simulink model "nivel3"  (R2018b)
settings: Solver=VariableStepAuto  StartTime=0.0  StopTime=10.0  RelTol=1e-3
libraries: fuzblock x3
settings Model: Creator=seba  LastModifiedBy=seba

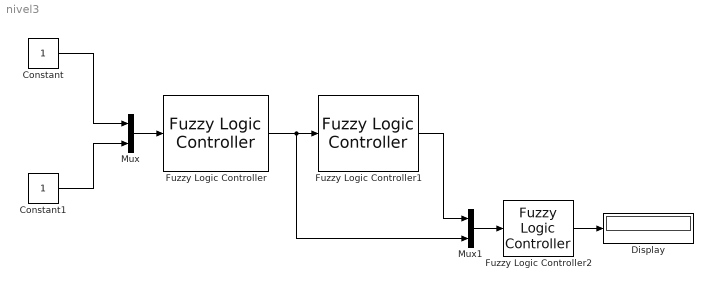
== system nivel3 ==
  Constant : Constant
  Constant1 : Constant
  Display : Display
      settings: Decimation=2
  Fuzzy Logic Controller : fuzblock/Fuzzy Logic  Controller  FIS=nivel1  OutputSampleNumber=101  DataType=double  FuzzifiedInputs=off  RuleFiringStrengths=off  RuleOutputs=off  AggregatedOutputs=off  SimulateUsing=Interpreted execution  OutOfRangeInputValueMessage=warning  NoRuleFiredMessage=warning  EmptyOutputFuzzySetMessage=warning
  Fuzzy Logic Controller1 : fuzblock/Fuzzy Logic  Controller  FIS=nivel2  OutputSampleNumber=101  DataType=double  FuzzifiedInputs=off  RuleFiringStrengths=off  RuleOutputs=off  AggregatedOutputs=off  SimulateUsing=Interpreted execution  OutOfRangeInputValueMessage=warning  NoRuleFiredMessage=warning  EmptyOutputFuzzySetMessage=warning
  Fuzzy Logic Controller2 : fuzblock/Fuzzy Logic  Controller  FIS=nivel3  OutputSampleNumber=101  DataType=double  FuzzifiedInputs=off  RuleFiringStrengths=off  RuleOutputs=off  AggregatedOutputs=off  SimulateUsing=Interpreted execution  OutOfRangeInputValueMessage=warning  NoRuleFiredMessage=warning  EmptyOutputFuzzySetMessage=warning
  Mux : Mux  Inputs=2
  Mux1 : Mux  Inputs=2
  wires:
  Mux/1 -> Fuzzy Logic Controller/1
  Constant/1 -> Mux/1
  Constant1/1 -> Mux/2
  Fuzzy Logic Controller/1 -> Mux1/2, Fuzzy Logic Controller1/1
  Mux1/1 -> Fuzzy Logic Controller2/1
  Fuzzy Logic Controller1/1 -> Mux1/1
  Fuzzy Logic Controller2/1 -> Display/1
